simulink model "retuning_controllers_v2"  (R2012b)
settings: Solver=ode45  StartTime=0.0  StopTime=10.0  RelTol=1e-3
libraries: fod x3
settings Model: Creator=Alex  LastModifiedBy=Alex

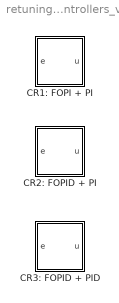
== system retuning_controllers_v2 ==
  CR1: FOPI + PI : Subsystem  mask{Kps=0.054972, Kis=0.055043, lambda=0.6631, Kp=0.0409, Ki=0.1229, Ts=0.001}
      mask prompts: Kps "Kp*"; Kis "Ki*"; Ts "Sampling interval"
  CR2: FOPID + PI : Subsystem  mask{Kps=0.005, Kis=0.021235, lambda=0.8, Kds=0.0014588, mu=0.5, Kp=0.0409, Ki=0.1229, Ts=0.001}
      mask prompts: Kps "Kp*"; Kis "Ki*"; Kds "Kd*"; Ts "Sampling interval"
  CR3: FOPID + PID : Subsystem  mask{Kps=0.005, Kis=0.021235, lambda=0.8, Kds=0.0014588, mu=0.5, Kp=0.0909, Ki=0.4546, Kd=0.0045, Ts=0.001}
      mask prompts: Kps "Kp*"; Kis "Ki*"; Kds "Kd*"; Ts "Sampling interval"

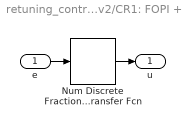
== system retuning_controllers_v2/CR1: FOPI + PI ==
  e : Inport
  Num Discrete Fractional Transfer Fcn : fod/Num Discrete Fractional Transfer Fcn  b=[Kis (Kps-Kp) -Ki]  nb=[1-lambda 1 0]  a=[Kp Ki]  na=[1 0]  freqRange=[0.001, 1000]  approxNum=5  useRef=off  dscrMethod=Matched  wc=0  ts=Ts
  u : Outport
  wires:
  e/1 -> Num Discrete Fractional Transfer Fcn/1
  Num Discrete Fractional Transfer Fcn/1 -> u/1

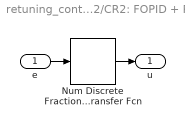
== system retuning_controllers_v2/CR2: FOPID + PI ==
  e : Inport
  Num Discrete Fractional Transfer Fcn : fod/Num Discrete Fractional Transfer Fcn  b=[Kds Kis (Kps-Kp) -Ki]  nb=[mu+1 1-lambda 1 0]  a=[Kp Ki]  na=[1 0]  freqRange=[0.001, 1000]  approxNum=5  useRef=off  dscrMethod=Matched  wc=0  ts=Ts
  u : Outport
  wires:
  Num Discrete Fractional Transfer Fcn/1 -> u/1
  e/1 -> Num Discrete Fractional Transfer Fcn/1

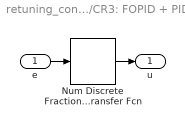
== system retuning_controllers_v2/CR3: FOPID + PID ==
  e : Inport
  Num Discrete Fractional Transfer Fcn : fod/Num Discrete Fractional Transfer Fcn  b=[Kds Kis -Kd (Kps-Kp) -Ki]  nb=[mu+1 1-lambda 2 1 0]  a=[Kd Kp Ki]  na=[2 1 0]  freqRange=[0.001, 1000]  approxNum=5  useRef=off  dscrMethod=Matched  wc=0  ts=Ts
  u : Outport
  wires:
  e/1 -> Num Discrete Fractional Transfer Fcn/1
  Num Discrete Fractional Transfer Fcn/1 -> u/1
